simulink model "ejh52"  (Simulink 3.00)
settings: Solver=ode45  StartTime=0.0  StopTime=10.0  RelTol=1e-3
libraries: HEMERO x2
settings Model: LastModifiedBy=Administrador

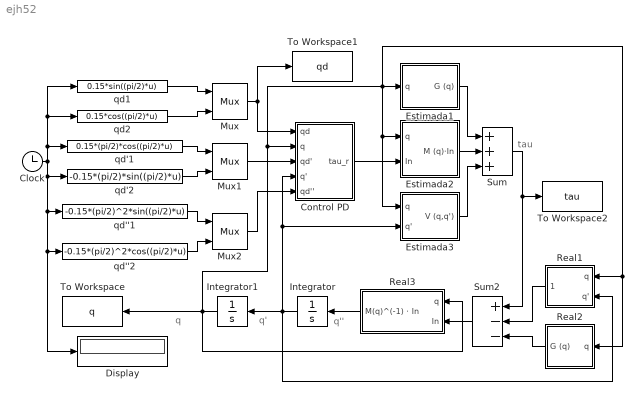
== system ejh52 ==
  note: tau
  note: q
  note: q'
  note: q''
  Clock : Clock
      settings: DisplayTime=off  Decimation=10
  Control PD : Subsystem  mask(Controlador PD){Kp=[25 0;0 25], Kv=[10 0;0 10]}
      mask prompts: Kp "Introduzca la matriz Kp:"; Kv "Introduzca la matriz Kv:"
      mask help: Calcula el par tau_r correspondiente a la técnica del par computado usando un controlador PD.
  Display : Display
      settings: Format=short
  Estimada1 : Subsystem  mask(Término gravitatorio){dyn=[0 0 0 0 0 2 3 0 0 0 0 0 0 0 0 0 1 0 0 0;0 3 0 0 0 1 1 0 0 0 0 0 0 0 0 0 1 0 0 0], grav=[0 -9.81 0]}
      mask prompts: dyn "Matriz de parámetros cinemáticos y dinámicos:"; grav "Vector aceleración de la gravedad:"
      mask help: Este bloque calcula el par correspondiente al término gravitatorio.
  Estimada2 : Subsystem  mask(Término asociado a la matriz de masas){dyn=[0 0 0 0 0 2 3 0 0 0 0 0 0 0 0 0 1 0 0 0;0 3 0 0 0 1 1 0 0 0 0 0 0 0 0 0 1 0 0 0]}
      mask prompts: dyn "Matriz de parámetros cinemáticos y dinámicos:"
      mask help: Este bloque calcula el par correspondiente al término en el que aparece la matriz de masas.
  Estimada3 : Subsystem  mask(Términos centrífugos y de Coriolis){dyn=[0 0 0 0 0 2 3 0 0 0 0 0 0 0 0 0 1 0 0 0;0 3 0 0 0 1 1 0 0 0 0 0 0 0 0 0 1 0 0 0]}
      mask prompts: dyn "Matriz de parámetros cinemáticos y dinámicos:"
      mask help: Este bloque calcula el par correspondiente a los términos centrífugos y de Coriolis.
  Integrator : Integrator  Orientation=left  ExternalReset=none  InitialConditionSource=internal  InitialCondition=[0;0]  LimitOutput=off  UpperSaturationLimit=inf  LowerSaturationLimit=-inf  ShowSaturationPort=off  ShowStatePort=off  AbsoluteTolerance=auto
  Integrator1 : Integrator  Orientation=left  ExternalReset=none  InitialConditionSource=internal  InitialCondition=[0; 0]  LimitOutput=off  UpperSaturationLimit=inf  LowerSaturationLimit=-inf  ShowSaturationPort=off  ShowStatePort=off  AbsoluteTolerance=auto
  Mux : Mux  Inputs=2
      settings: DisplayOption=none
  Mux1 : Mux  Inputs=2
      settings: DisplayOption=none
  Mux2 : Mux  Inputs=2
      settings: DisplayOption=none
  Real1 : Subsystem  Orientation=left  mask(Términos centrífugos y de Coriolis){dyn=[0 0 0 0 0 2 3 0 0 0 0 0 0 0 0 0 1 0 0 0;0 3 0 0 0 1 1 0 0 0 0 0 0 0 0 0 1 0 0 0]}
      mask prompts: dyn "Matriz de parámetros cinemáticos y dinámicos:"
      mask help: Este bloque calcula el par correspondiente a los términos centrífugos y de Coriolis.
  Real2 : Subsystem  Orientation=left  mask(Término gravitatorio){dyn=[0 0 0 0 0 2 3 0 0 0 0 0 0 0 0 0 1 0 0 0;0 3 0 0 0 1 1 0 0 0 0 0 0 0 0 0 1 0 0 0], grav=[0 -9.81 0]}
      mask prompts: dyn "Matriz de parámetros cinemáticos y dinámicos:"; grav "Vector aceleración de la gravedad:"
      mask help: Este bloque calcula el par correspondiente al término gravitatorio.
  Real3 : Subsystem  Orientation=left  mask(Inversa de la matriz de masas){dyn=[0 0 0 0 0 2 3 0 0 0 0 0 0 0 0 0 1 0 0 0;0 3 0 0 0 1 1 0 0 0 0 0 0 0 0 0 1 0 0 0]}
      mask prompts: dyn "Matriz de parámetros cinemáticos y dinámicos:"
      mask help: Este bloque calcula el producto de la inversa de la matriz de masas por el vector columna In que se le pasa como entrada.
  Sum : Sum  Inputs=+++  SaturateOnIntegerOverflow=on
  Sum2 : Sum  Orientation=left  Inputs=+--  SaturateOnIntegerOverflow=on
  To Workspace : ToWorkspace  VariableName=q  SampleTime=-1  SaveFormat=Matrix
  To Workspace1 : ToWorkspace  VariableName=qd  SampleTime=-1  SaveFormat=Matrix
  To Workspace2 : ToWorkspace  VariableName=tau  SampleTime=-1  SaveFormat=Matrix
  qd''1 : Fcn  Expr=-0.15*(pi/2)^2*sin((pi/2)*u)
  qd''2 : Fcn  Expr=-0.15*(pi/2)^2*cos((pi/2)*u)
  qd'1 : Fcn  Expr=0.15*(pi/2)*cos((pi/2)*u)
  qd'2 : Fcn  Expr=-0.15*(pi/2)*sin((pi/2)*u)
  qd1 : Fcn  Expr=0.15*sin((pi/2)*u)
  qd2 : Fcn  Expr=0.15*cos((pi/2)*u)
  wires:
  Sum/1 -> To Workspace2/1, Sum2/1
  Mux/1 -> To Workspace1/1, Control PD/1(qd)
  Control PD/1(tau_r) -> Estimada2/2(In)
  Clock/1 -> qd'1/1, qd2/1, qd1/1, qd'2/1, qd''1/1, qd''2/1, Display/1
  qd1/1 -> Mux/1
  qd2/1 -> Mux/2
  qd'1/1 -> Mux1/1
  qd'2/1 -> Mux1/2
  qd''1/1 -> Mux2/1
  qd''2/1 -> Mux2/2
  Mux1/1 -> Control PD/3(qd')
  Mux2/1 -> Control PD/5(qd'')
  Estimada2/1(M (q)·In) -> Sum/2
  Estimada1/1(G (q)) -> Sum/1
  Estimada3/1(V (q,q')) -> Sum/3
  Real2/1(G (q)) -> Sum2/3
  Real1/1(V (q,q')) -> Sum2/2
  Sum2/1 -> Real3/2(In)
  Integrator/1 -> Integrator1/1, Control PD/4(q'), Estimada3/2(q'), Real1/2(q')
  Integrator1/1 -> Control PD/2(q), Estimada1/1(q), Estimada2/1(q), Estimada3/1(q), Real1/1(q), Real2/1(q), To Workspace/1, Real3/1(q)
  Real3/1(M(q)^(-1) · In) -> Integrator/1

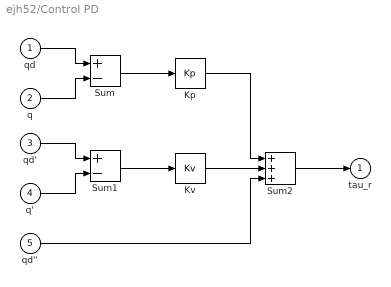
== system ejh52/Control PD ==
  qd : Inport  Port=1  PortWidth=-1  SampleTime=-1  DataType=auto
      settings: SignalType=auto
  q : Inport  Port=2  PortWidth=-1  SampleTime=-1  DataType=auto
      settings: SignalType=auto
  qd' : Inport  Port=3  PortWidth=-1  SampleTime=-1  DataType=auto
      settings: SignalType=auto
  q' : Inport  Port=4  PortWidth=-1  SampleTime=-1  DataType=auto
      settings: SignalType=auto
  qd'' : Inport  Port=5  PortWidth=-1  SampleTime=-1  DataType=auto
      settings: SignalType=auto
  Kp : HEMERO/Robots manipuladores base fija/Control basado en el modelo/Par Computado/Ejemplos/Ejemplo H.5.2/Control PD/Kp  MaskParam1=Kp
  Kv : HEMERO/Robots manipuladores base fija/Control basado en el modelo/Par Computado/Ejemplos/Ejemplo H.5.2/Control PD/Kv  MaskParam1=Kv
  Sum : Sum  Inputs=+-  SaturateOnIntegerOverflow=on
  Sum1 : Sum  Inputs=+-  SaturateOnIntegerOverflow=on
  Sum2 : Sum  Inputs=+++  SaturateOnIntegerOverflow=on
  tau_r : Outport  Port=1  InitialOutput=0
  wires:
  qd/1 -> Sum/1
  q/1 -> Sum/2
  qd'/1 -> Sum1/1
  q'/1 -> Sum1/2
  Sum/1 -> Kp/1
  Sum1/1 -> Kv/1
  Kv/1 -> Sum2/2
  Kp/1 -> Sum2/1
  qd''/1 -> Sum2/3
  Sum2/1 -> tau_r/1

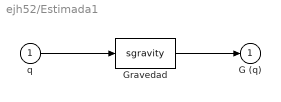
== system ejh52/Estimada1 ==
  q : Inport  Port=1  PortWidth=-1  SampleTime=-1  DataType=auto
      settings: SignalType=auto
  Gravedad : S-Function  FunctionName=sgravity  Parameters=dyn,grav  PortCounts=[]  SFunctionModules=''
  G (q) : Outport  Port=1  InitialOutput=0
  wires:
  q/1 -> Gravedad/1
  Gravedad/1 -> G (q)/1

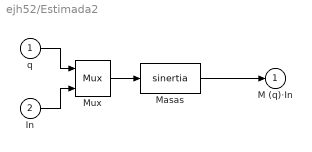
== system ejh52/Estimada2 ==
  q : Inport  Port=1  PortWidth=-1  SampleTime=-1  DataType=auto
      settings: SignalType=auto
  In : Inport  Port=2  PortWidth=-1  SampleTime=-1  DataType=auto
      settings: SignalType=auto
  Masas : S-Function  FunctionName=sinertia  Parameters=dyn  PortCounts=[]  SFunctionModules=''
  Mux : Mux  Inputs=2
      settings: DisplayOption=none
  M (q)·In : Outport  Port=1  InitialOutput=0
  wires:
  Mux/1 -> Masas/1
  q/1 -> Mux/1
  In/1 -> Mux/2
  Masas/1 -> M (q)·In/1

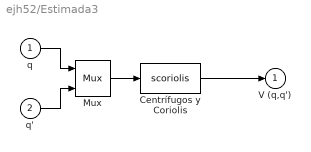
== system ejh52/Estimada3 ==
  q : Inport  Port=1  PortWidth=-1  SampleTime=-1  DataType=auto
      settings: SignalType=auto
  q' : Inport  Port=2  PortWidth=-1  SampleTime=-1  DataType=auto
      settings: SignalType=auto
  Centrífugos y Coriolis : S-Function  FunctionName=scoriolis  Parameters=dyn  PortCounts=[]  SFunctionModules=''
  Mux : Mux  Inputs=2
      settings: DisplayOption=none
  V (q,q') : Outport  Port=1  InitialOutput=0
  wires:
  Mux/1 -> Centrífugos y Coriolis/1
  q/1 -> Mux/1
  q'/1 -> Mux/2
  Centrífugos y Coriolis/1 -> V (q,q')/1

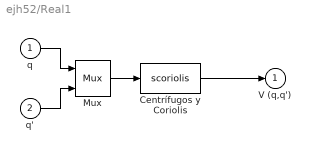
== system ejh52/Real1 ==
  q : Inport  Port=1  PortWidth=-1  SampleTime=-1  DataType=auto
      settings: SignalType=auto
  q' : Inport  Port=2  PortWidth=-1  SampleTime=-1  DataType=auto
      settings: SignalType=auto
  Centrífugos y Coriolis : S-Function  FunctionName=scoriolis  Parameters=dyn  PortCounts=[]  SFunctionModules=''
  Mux : Mux  Inputs=2
      settings: DisplayOption=none
  V (q,q') : Outport  Port=1  InitialOutput=0
  wires:
  Mux/1 -> Centrífugos y Coriolis/1
  q/1 -> Mux/1
  q'/1 -> Mux/2
  Centrífugos y Coriolis/1 -> V (q,q')/1

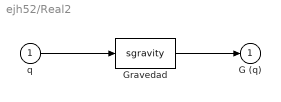
== system ejh52/Real2 ==
  q : Inport  Port=1  PortWidth=-1  SampleTime=-1  DataType=auto
      settings: SignalType=auto
  Gravedad : S-Function  FunctionName=sgravity  Parameters=dyn,grav  PortCounts=[]  SFunctionModules=''
  G (q) : Outport  Port=1  InitialOutput=0
  wires:
  q/1 -> Gravedad/1
  Gravedad/1 -> G (q)/1

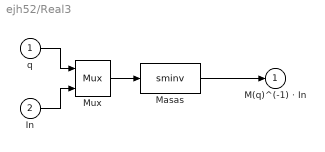
== system ejh52/Real3 ==
  q : Inport  Port=1  PortWidth=-1  SampleTime=-1  DataType=auto
      settings: SignalType=auto
  In : Inport  Port=2  PortWidth=-1  SampleTime=-1  DataType=auto
      settings: SignalType=auto
  Masas : S-Function  FunctionName=sminv  Parameters=dyn  PortCounts=[]  SFunctionModules=''
  Mux : Mux  Inputs=2
      settings: DisplayOption=none
  M(q)^(-1) · In : Outport  Port=1  InitialOutput=0
  wires:
  Mux/1 -> Masas/1
  q/1 -> Mux/1
  In/1 -> Mux/2
  Masas/1 -> M(q)^(-1) · In/1
